simulink model "projet"  (R2023a)
settings: Solver=VariableStepAuto  StartTime=0.0  StopTime=100  RelTol=1e-3
values from neighbouring files (symbols this model uses):
  a = 0.102    [initiation.m]
  b = 0    [initiation.m]
  c = 0.5    [initiation.m]
  d = 3    [Robot.m]    (also in initiation.m = 1)
  f = 0.1    [initiation.m]
  K_delta = -1    [initiation.m]
  Kp = 5    [initiation.m]
  rayon = 2    [initiation.m]
  theta0 = 0    [initiation.m]
  x0 = 1    [initiation.m]
  y0 = 1.5    [initiation.m]
settings Model: Creator=Lelhadi2022  LastModifiedBy=Lelhadi2022

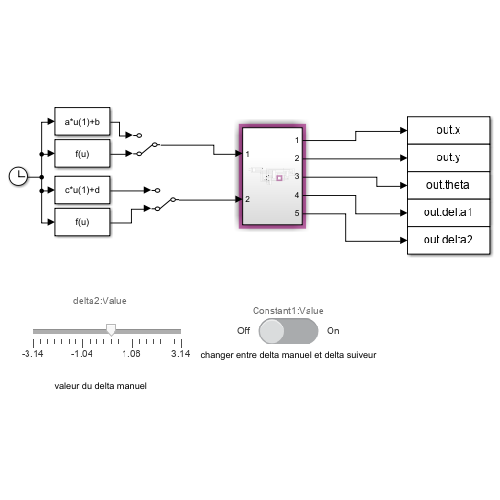
[thumbnail: Simulink's stored preview of the top-level diagram]
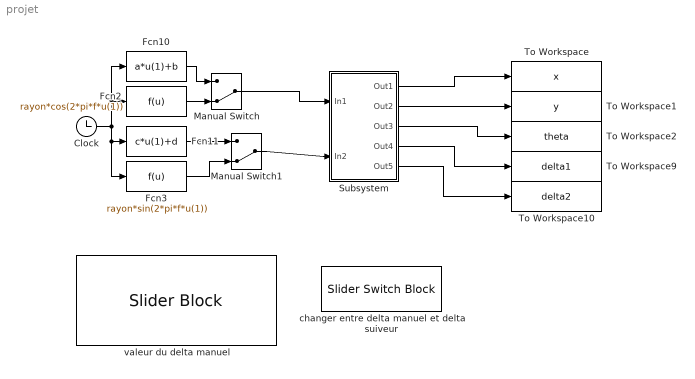
== system projet ==
  Clock : Clock
  Fcn10 : Fcn  Expr=a*u(1)+b
  Fcn11 : Fcn  Expr=c*u(1)+d
  Fcn2 : Fcn  Expr=rayon*cos(2*pi*f*u(1))
  Fcn3 : Fcn  Expr=rayon*sin(2*pi*f*u(1))
  Manual Switch : ManualSwitch  CurrentSetting=0
  Manual Switch1 : ManualSwitch  CurrentSetting=0
  Subsystem : Subsystem
  To Workspace : ToWorkspace  VariableName=x  SaveFormat=Timeseries  SampleTime=-1
  To Workspace1 : ToWorkspace  VariableName=y  SaveFormat=Timeseries  SampleTime=-1
  To Workspace10 : ToWorkspace  VariableName=delta2  SaveFormat=Timeseries  SampleTime=-1
  To Workspace2 : ToWorkspace  VariableName=theta  SaveFormat=Timeseries  SampleTime=-1
  To Workspace9 : ToWorkspace  VariableName=delta1  SaveFormat=Timeseries  SampleTime=-1
  changer entre delta manuel et delta suiveur : SliderSwitchBlock
      settings: Values={{'Off', 'On'}, [0 1]}
  valeur du delta manuel : SliderBlock  ScaleMin=-3.14  ScaleMax=3.14
  wires:
  Clock/1 -> Fcn11/1, Fcn3/1, Fcn10/1, Fcn2/1
  Fcn2/1 -> Manual Switch/2
  Fcn3/1 -> Manual Switch1/2
  Fcn10/1 -> Manual Switch/1
  Fcn11/1 -> Manual Switch1/1
  Manual Switch/1 -> Subsystem/1(In1)
  Manual Switch1/1 -> Subsystem/2(In2)
  Subsystem/1(Out1) -> To Workspace/1
  Subsystem/2(Out2) -> To Workspace1/1
  Subsystem/3(Out3) -> To Workspace2/1
  Subsystem/4(Out4) -> To Workspace9/1
  Subsystem/5(Out5) -> To Workspace10/1

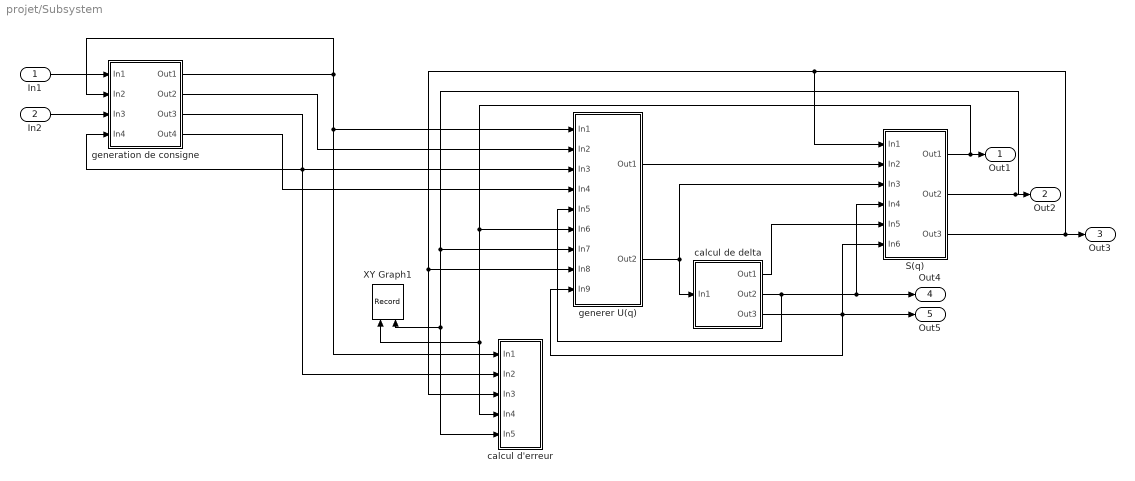
== system projet/Subsystem ==
  In1 : Inport
  In2 : Inport  Port=2
  S(q) : Subsystem
  XY Graph1 : Record  FileSettingsInternal="{\"entries\":[{\"content\":{\"excelSettings\":{\"content\":{},\"type\":\"Streamout.ExcelSettings\"}},\"type\":\"Streamout.FileSettingStorage\",\"uuid\":\"\"}],\"packageUris\":[\"http:\\/\\/schema.mathworks.com\\/mf0\\/streamout_blocks\\/R2020a\"],\"version\":\"1.0\"}"  Layout=[1 1]  SignalsInternal="{\"entries\":[{\"content\":{\"signals\":[{\"content\":{\"blockPath\":[],\"dimensions\":[1],\"domain\":\"\",\"lineColor\":\"#0072bd\",\"port\":1,\"sid\":[\"\"],\"signalID\":192,\"signalName\":\"S(q):1\"},\"type\":\"RecordBlkView.Signal\",\"uuid\":\"\"},{\"content\":{\"blockPath\":[],\"dimensions\":[1],\"domain\":\"\",\"lineColor\":\"#d95319\",\"port\":2,\"sid\":[\"\"],\"signalID\":196,\"signalName\":\"S(q):2\"},\"type\":\"RecordBlkView.Signal\",\"uuid\":\"\"}]},\"type\":\"RecordBlkView.InputSignals\",\"uuid\":\"\"}],\"packageUris\":[\"http:\\/\\/schema.mathworks.com\\/mf0\\/streamout_blocks\\/R2020a\"],\"version\":\"1.0\"}"  VisualizationBindings="{\"xyplotplugin\":{\"info\":[{\"series\":[{\"bindingParametersList\":[{\"parameter\":\"X-Axis\",\"signalID\":43,\"signalName\":\"Integrator1\"},{\"parameter\":\"Y-Axis\",\"signalID\":47,\"signalName\":\"Integrator5\"}],\"seriesID\":48808}],\"subplotID\":1}]}}"  CompatibilityTag=XY
  calcul d'erreur : Subsystem
  "calcul de delta " : Subsystem
  generation de consigne : Subsystem
  generer U(q) : Subsystem
  Out1 : Outport
  Out2 : Outport  Port=2
  Out3 : Outport  Port=3
  Out4 : Outport  Port=4
  Out5 : Outport  Port=5
  wires:
  "calcul de delta "/2(Out2) -> S(q)/4(In4), Out4/1, generer U(q)/5(In5)
  "calcul de delta "/3(Out3) -> generer U(q)/9(In9), Out5/1, S(q)/6(In6)
  S(q)/1(Out1) -> Out1/1, generer U(q)/6(In6), XY Graph1/1, calcul d'erreur/4(In4)
  S(q)/2(Out2) -> generer U(q)/7(In7), XY Graph1/2, calcul d'erreur/5(In5), Out2/1
  S(q)/3(Out3) -> Out3/1, S(q)/1(In1), calcul d'erreur/3(In3), generer U(q)/8(In8)
  "calcul de delta "/1(Out1) -> S(q)/5(In5)
  generer U(q)/2(Out2) -> S(q)/3(In3), "calcul de delta "/1(In1)
  generer U(q)/1(Out1) -> S(q)/2(In2)
  generation de consigne/1(Out1) -> calcul d'erreur/1(In1), generer U(q)/1(In1), generation de consigne/2(In2)
  generation de consigne/3(Out3) -> generation de consigne/4(In4), calcul d'erreur/2(In2), generer U(q)/3(In3)
  In1/1 -> generation de consigne/1(In1)
  In2/1 -> generation de consigne/3(In3)
  generation de consigne/2(Out2) -> generer U(q)/2(In2)
  generation de consigne/4(Out4) -> generer U(q)/4(In4)

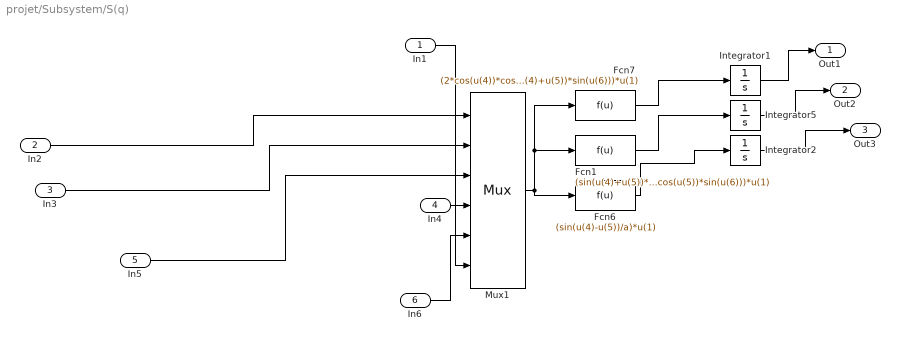
== system projet/Subsystem/S(q) ==
  In1 : Inport
  In2 : Inport  Port=2
  In3 : Inport  Port=3
  In4 : Inport  Port=4
  In5 : Inport  Port=5
  In6 : Inport  Port=6
  Fcn1 : Fcn  Expr=(sin(u(4)+u(5))*cos(u(6))+2*cos(u(4))*cos(u(5))*sin(u(6)))*u(1)
  Fcn6 : Fcn  Expr=(sin(u(4)-u(5))/a)*u(1)
  Fcn7 : Fcn  Expr=(2*cos(u(4))*cos(u(5))*cos(u(6))-sin(u(4)+u(5))*sin(u(6)))*u(1)
  Integrator1 : Integrator  InitialCondition=x0
  Integrator2 : Integrator  InitialCondition=theta0
  Integrator5 : Integrator  InitialCondition=y0
  Mux1 : Mux  Inputs=6
  Out1 : Outport
  Out2 : Outport  Port=2
  Out3 : Outport  Port=3
  wires:
  Mux1/1 -> Fcn7/1, Fcn1/1, Fcn6/1
  In6/1 -> Mux1/5
  Fcn6/1 -> Integrator2/1
  In4/1 -> Mux1/4
  Fcn1/1 -> Integrator5/1
  Integrator2/1 -> Out3/1
  Integrator5/1 -> Out2/1
  Integrator1/1 -> Out1/1
  Fcn7/1 -> Integrator1/1
  In3/1 -> Mux1/2
  In2/1 -> Mux1/1
  In1/1 -> Mux1/6
  In5/1 -> Mux1/3

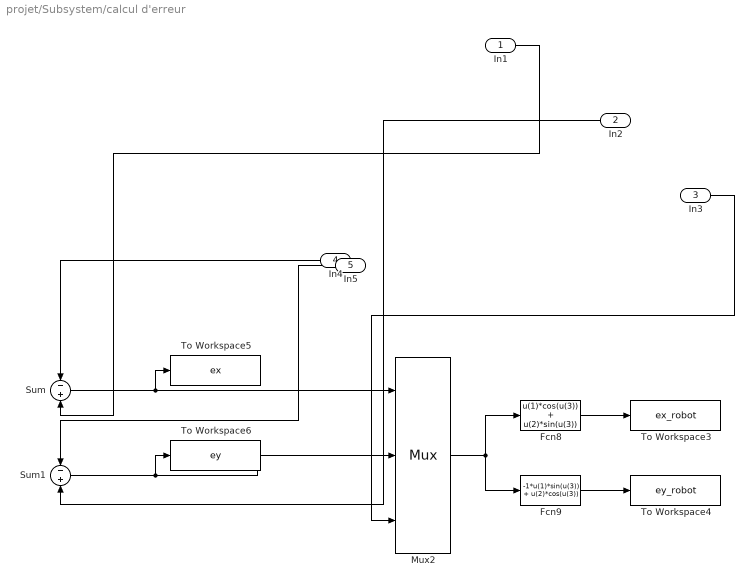
== system projet/Subsystem/calcul d'erreur ==
  In1 : Inport
  In2 : Inport  Port=2
  In3 : Inport  Port=3
  In4 : Inport  Port=4
  In5 : Inport  Port=5
  Fcn8 : Fcn  Expr=u(1)*cos(u(3)) + u(2)*sin(u(3))
  Fcn9 : Fcn  Expr=-1*u(1)*sin(u(3)) + u(2)*cos(u(3))
  Mux2 : Mux  Inputs=3
  Sum : Sum  Inputs=-|+
  Sum1 : Sum  Inputs=-|+
  To Workspace3 : ToWorkspace  VariableName=ex_robot  SaveFormat=Timeseries  SampleTime=-1
  To Workspace4 : ToWorkspace  VariableName=ey_robot  SaveFormat=Timeseries  SampleTime=-1
  To Workspace5 : ToWorkspace  VariableName=ex  SaveFormat=Timeseries  SampleTime=-1
  To Workspace6 : ToWorkspace  VariableName=ey  SaveFormat=Timeseries  SampleTime=-1
  wires:
  Mux2/1 -> Fcn9/1, Fcn8/1
  Fcn9/1 -> To Workspace4/1
  In5/1 -> Sum1/1
  In3/1 -> Mux2/3
  Sum1/1 -> To Workspace6/1, Mux2/2
  Sum/1 -> To Workspace5/1, Mux2/1
  In1/1 -> Sum/2
  Fcn8/1 -> To Workspace3/1
  In2/1 -> Sum1/2
  In4/1 -> Sum/1

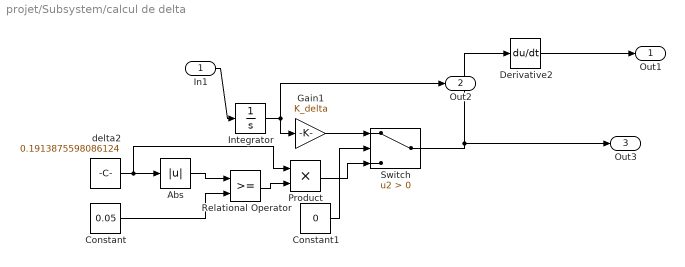
== system projet/Subsystem/calcul de delta  ==
  In1 : Inport
  Abs : Abs  SaturateOnIntegerOverflow=off
  Constant : Constant  Value=0.05
  Constant1 : Constant  Value=0
  Derivative2 : Derivative
  Gain1 : Gain  Gain=K_delta
  Integrator : Integrator
  Product : Product
  Relational Operator : RelationalOperator  OutDataTypeStr=boolean  RndMeth=Simplest  InputSameDT=off
  Switch : Switch  Criteria=u2 > Threshold  SaturateOnIntegerOverflow=off  InputSameDT=off
  delta2 : Constant  Value=0.1913875598086124
  Out1 : Outport
  Out2 : Outport  Port=2
  Out3 : Outport  Port=3
  wires:
  Switch/1 -> Out3/1, Derivative2/1
  Relational Operator/1 -> Product/2
  Gain1/1 -> Switch/1
  Constant/1 -> Relational Operator/2
  In1/1 -> Integrator/1
  delta2/1 -> Product/1, Abs/1
  Integrator/1 -> Out2/1, Gain1/1
  Abs/1 -> Relational Operator/1
  Constant1/1 -> Switch/2
  Product/1 -> Switch/3
  Derivative2/1 -> Out1/1

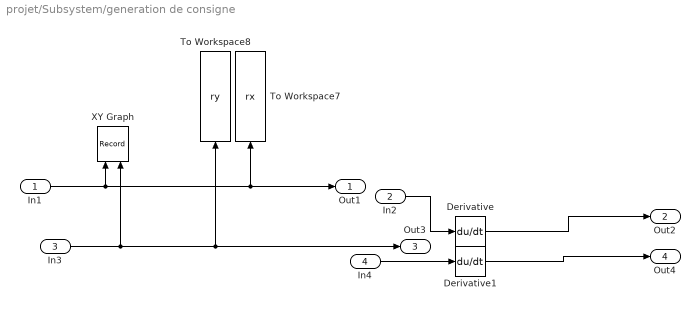
== system projet/Subsystem/generation de consigne ==
  In1 : Inport
  In2 : Inport  Port=2
  In3 : Inport  Port=3
  In4 : Inport  Port=4
  Derivative : Derivative
  Derivative1 : Derivative
  To Workspace7 : ToWorkspace  VariableName=rx  SaveFormat=Timeseries  SampleTime=-1
  To Workspace8 : ToWorkspace  VariableName=ry  SaveFormat=Timeseries  SampleTime=-1
  XY Graph : Record  FileSettingsInternal="{\"entries\":[{\"content\":{\"excelSettings\":{\"content\":{},\"type\":\"Streamout.ExcelSettings\"}},\"type\":\"Streamout.FileSettingStorage\",\"uuid\":\"\"}],\"packageUris\":[\"http:\\/\\/schema.mathworks.com\\/mf0\\/streamout_blocks\\/R2020a\"],\"version\":\"1.0\"}"  Layout=[1 1]  SignalsInternal="{\"entries\":[{\"content\":{\"signals\":[{\"content\":{\"blockPath\":[],\"dimensions\":[1],\"domain\":\"\",\"lineColor\":\"#a2142f\",\"port\":1,\"sid\":[\"\"],\"signalID\":216,\"signalName\":\"In1\"},\"type\":\"RecordBlkView.Signal\",\"uuid\":\"\"},{\"content\":{\"blockPath\":[],\"dimensions\":[1],\"domain\":\"\",\"lineColor\":\"#139fff\",\"port\":2,\"sid\":[\"\"],\"signalID\":220,\"signalName\":\"In3\"},\"type\":\"RecordBlkView.Signal\",\"uuid\":\"\"}]},\"type\":\"RecordBlkView.InputSignals\",\"uuid\":\"\"}],\"packageUris\":[\"http:\\/\\/schema.mathworks.com\\/mf0\\/streamout_blocks\\/R2020a\"],\"version\":\"1.0\"}"  VisualizationBindings="{\"xyplotplugin\":{\"info\":[{\"series\":[{\"bindingParametersList\":[{\"parameter\":\"X-Axis\",\"signalID\":35,\"signalName\":\"Manual Switch\"},{\"parameter\":\"Y-Axis\",\"signalID\":39,\"signalName\":\"Manual Switch1\"}],\"seriesID\":33380}],\"subplotID\":1}]}}"  CompatibilityTag=XY
  Out1 : Outport
  Out2 : Outport  Port=2
  Out3 : Outport  Port=3
  Out4 : Outport  Port=4
  wires:
  In3/1 -> Out3/1, To Workspace8/1, XY Graph/2
  In2/1 -> Derivative/1
  In1/1 -> Out1/1, To Workspace7/1, XY Graph/1
  In4/1 -> Derivative1/1
  Derivative/1 -> Out2/1
  Derivative1/1 -> Out4/1

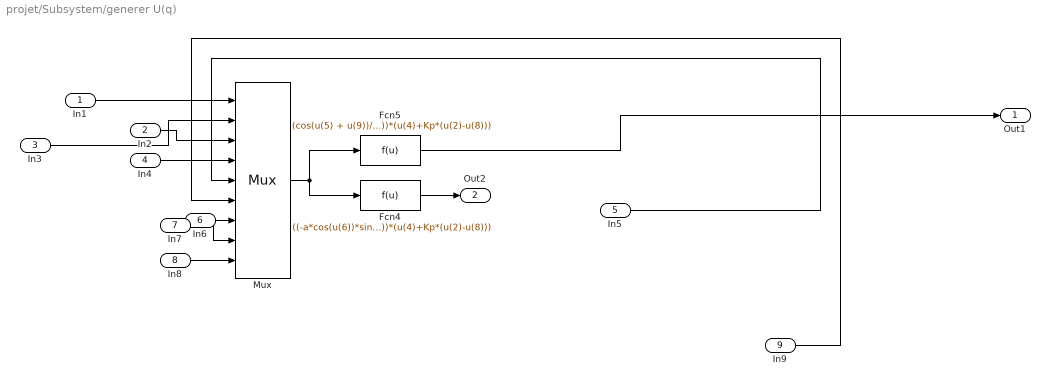
== system projet/Subsystem/generer U(q) ==
  In1 : Inport
  In2 : Inport  Port=2
  In3 : Inport  Port=3
  In4 : Inport  Port=4
  In5 : Inport  Port=5
  In6 : Inport  Port=6
  In7 : Inport  Port=7
  In8 : Inport  Port=8
  In9 : Inport  Port=9
  Fcn4 : Fcn  Expr=((-a*cos(u(6))*sin(u(5)+u(9))-e*sin(u(5)-u(6))*cos(u(5)+u(9)))/(a*e*sin(u(5) + u(9))^2*cos(u(6)) + a*e*cos(u(6))*cos(u(5)+u(9))^2))*(u(3)+Kp*(u(1)-u(7)))+((a*cos(u(6))*cos(u(5)+u(9))-e*sin(u(5)-u(6))*sin(u(5)+u(9)))/(a*e*sin(u(5) + u(9))^2*cos(u(6)) + a*e*cos(u(6))*cos(u(5)+u(9))^2))*(u(4)+Kp*(u(2)-u(8)))
  Fcn5 : Fcn  Expr=(cos(u(5) + u(9))/(2*sin(u(5) + u(9))^2*cos(u(6)) + 2*cos(u(6))*cos(u(5) + u(9))^2))*(u(3)+Kp*(u(1)-u(7)))+(sin(u(5) +u(9))/(2*sin(u(5) + u(9))^2*cos(u(6))+2*cos(u(6))*cos(u(5)+u(9))^2))*(u(4)+Kp*(u(2)-u(8)))
  Mux : Mux  Inputs=9
  Out1 : Outport
  Out2 : Outport  Port=2
  wires:
  In3/1 -> Mux/2
  In5/1 -> Mux/5
  Mux/1 -> Fcn5/1, Fcn4/1
  In1/1 -> Mux/1
  Fcn5/1 -> Out1/1
  In7/1 -> Mux/8
  In9/1 -> Mux/6
  In4/1 -> Mux/4
  In2/1 -> Mux/3
  Fcn4/1 -> Out2/1
  In6/1 -> Mux/7
  In8/1 -> Mux/9
